simulink model "FIR_TDM_Ex2"  (R2023a)
settings: Solver=VariableStepAuto  StartTime=0.0  StopTime=5  RelTol=1e-3
InitFcn:
  | NumOf_TDM_Channels = 8;
  | SamplesPerChannel = 128;
  | FilterLength = 16;
  | f = dsp.Channelizer(NumOf_TDM_Channels,1,Specification="coefficients");
  | blowpass = firpm(FilterLength-1,[0 .2 .4 1],[1 1 0 0]);
  | N = length(blowpass)-1;
  | Fc = 0.4;
  | j = complex(0,1);
  | bbandpass = blowpass.*exp(j*Fc*pi*(0:N));
  | f.LowpassCoefficients = bbandpass;
  | f.freqz
  | filters = f.getFilters;
  | filters = round(filters, 14, TieBreaker="fromzero");
undefined symbols (not defined in the file): Asymmetric, S, vsva2197, xcvc1902
libraries: aieUtilities x3, dspsrcs4 x2, aieDSP x1, vmcUtilities x1
settings Model: Creator=sdegala  LastModifiedBy=sdegala

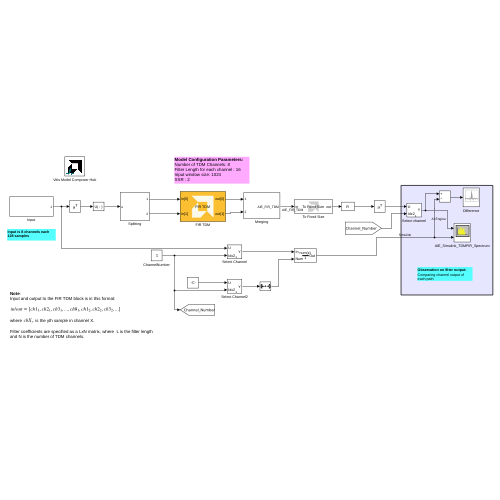
[thumbnail: Simulink's stored preview of the top-level diagram]
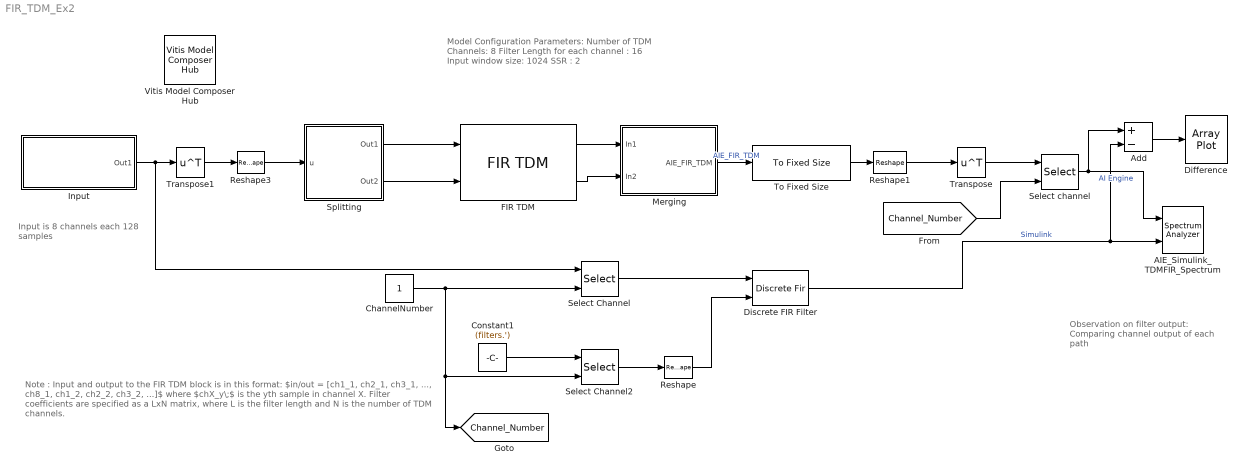
== system FIR_TDM_Ex2 ==
  note: Observation on filter output:
      | Comparing channel output of each path
  note: Input is 8 channels each 128 samples
  note: Model Configuration Parameters:
      | Number of TDM Channels: 8
      | Filter Length for each channel : 16
      | Input window size: 1024
      | SSR : 2
  note: Note :
      | Input and output to the FIR TDM block is in this format:
      |
      | $in/out = [ch1_1, ch2_1, ch3_1, ..., ch8_1, ch1_2, ch2_2, ch3_2, ...]$
      |
      | where $chX_y\;$ is the yth sample in channel X.
      |
      | Filter coefficients are specified as a LxN matrix, where L is the filter length and N is the number of TDM channels.
  AIE_Simulink_TDMFIR_Spectrum : SpectrumAnalyzer  NumInputPorts=2  WindowPosition=[265.000000,-185.000000,936.000000,716.000000,]  Visible=on  ScopeFrameLocation=window  Span=12499.999999999998  StartFrequency=-6249.999999999999  StopFrequency=6249.999999999999  YLimits=[-92.75639585,-29.1140143]  ShowLegend=on  SelectedToolstripTab=spectrumAnalyzerToolstrip.channelMeasurementsTab  MeasurementChannel=2
  Add : Sum  Inputs=+-
  ChannelNumber : Constant  OutDataTypeStr=uint16  SampleTime=-1
  Constant1 : Constant  Value=(filters.')  OutDataTypeStr=single  SampleTime=-1
  Difference : ArrayPlot  WindowPosition=[349.000000,17.000000,800.000000,500.000000,]  Visible=on  ScopeFrameLocation=window  XDataMode=Custom  XOffset=[-0.5 0.5]  PlotType=Line  AxesScaling=Manual  YLimits=[-0.5 0.5]  ShowLegend=on
  Discrete FIR Filter : DiscreteFir  CoefSource=Input port  Coefficients=filters(1,:)  InputProcessing=Columns as channels (frame based)  RndMeth=Round
      settings: InputPortMap=u0,u1
  FIR TDM : aieDSP/FIR TDM  data_type=cfloat  data_out_type=cfloat  coef_type=cfloat  fir_length=FilterLength  coeff=(filters.')  shift_val=0  rnd_mode=Floor  input_window_size=NumOf_TDM_Channels*SamplesPerChannel  tdm_channels=NumOf_TDM_Channels  sat_mode=1-Asymmetric  casc_length=1  ssr=2  AIE_VARIANT=1  blockJsonConstraints=[]  blockJsonConstraintsInternal=[]  spec=vmc_fir_tdm.json  SerializedMaskParamNames=[]  SerializedMaskParamValues=[]  SerializedMaskParamVisibilities=[]  block_type=FIR TDM  SerializedMaskParamDataypes=typename|typename|typename|uint|coef_type|uint|uint|uint|uint|uint|uint|uint|uint  SerializedMaskParamEnumStrArr=0|0|0|0|0|0|Floor,Ceiling,Round to positive infinity,Round to negative infinity,Round symmetrical to infinity,Round symmetrical to zero,Round convergent to even,Round convergent to odd|0|0|0-None,1-Asymmetric,3-Symmetric|0|0|0  SerializedMaskParamEnumValArr=0|0|0|0|0|0|0,1,2,3,4,5,6,7|0|0|0,1,3|0|0|0  SerializedMaskParamVectorArr=0|0|0|0|1|0|0|0|0|0|0|0|0
  Input : Subsystem
  Merging : Subsystem
  Reshape : Reshape  OutputDimensionality=Row vector (2-D)
  Reshape1 : Reshape  OutputDimensionality=Customize  OutputDimensions=[NumOf_TDM_Channels,SamplesPerChannel]
  Reshape3 : Reshape
  Select Channel : Selector  NumberOfDimensions=2  InputPortWidth=3  IndexOptions=Select all,Index vector (port)  Indices=3,[16]  OutputSizes=1,1
  Select Channel2 : Selector  NumberOfDimensions=2  InputPortWidth=3  IndexOptions=Select all,Index vector (port)  Indices=3,[16]  OutputSizes=1,1
  Select channel : Selector  NumberOfDimensions=2  InputPortWidth=3  IndexOptions=Select all,Index vector (port)  Indices=3,[16]  OutputSizes=1,1
  Splitting : Subsystem
  To Fixed Size : aieUtilities/To Fixed Size  Mode=Stop simulation when input variable-size signal is not full  OutputSize=Inherit: Same as input  CopyMethod=Buffer samples to form output  HasStatusOutput=on
  Transpose : Math  Operator=transpose
  Transpose1 : Math  Operator=transpose
  Vitis Model Composer Hub : vmcUtilities/Vitis Model Composer Hub  Tag=genX  CodeGeneration=off  StartColumn=1  NumberOfColumns=1  TargetDirectory=./code  exportDesign=off  analyzeDesign=off  validateDesignOnHw=off  ExportType=AI Engines  IpVendor=xilinx.com  IpLibrary=hls  IpVersion=1.0  IpHWLanguage=Verilog  AieCompilerOptions={}  AieSimulatorOptions={}  CreateTestbench=off  TestbenchStackSize=10  RunRtlSim=off  RunCSim=off  RunAieSim=off  AieSimTimeout=50000  RunAieSimProfiling=off  LaunchVitisAnalyzer=off  PlotOutput=off  RunX86Sim=off  X86SimTimeout=10  GenHwImage=off  GenLibadfXo=off  GenHwValidationCode=off  PlatformType=Not Specified  HwSystemType=Baremetal  HwValidationTarget=hw  ProjDevice=xcvc1902-vsva2197-1LP-e-S  ProjDevicePart=xcvc1902-vsva2197-1LP-e-S  AIEType=AIE  SamplePeriod=-1  ClockFrequency=200  DataPathParallelism=1  xilinxfamily=versalaicore  part=xcvc1902  speed=-1LP-e-S  package=vsva2197  directory=./netlist  testbench=off  incr_netlist=off  synthesis_tool=Vivado  clock_wrapper=Clock Enables  dbl_ovrd=According to Block Masks  dcm_input_clock_period=10  sysclk_period=10  simulink_period=1  eval_field=0  LogFileName=''  NThreads=4
  tag scope: Channel_Number=global
  wires:
  Reshape1/1 -> Transpose/1
  Select channel/1 -> Add/1, AIE_Simulink_TDMFIR_Spectrum/1  "AI Engine"
  Transpose1/1 -> Reshape3/1
  Transpose/1 -> Select channel/1
  Input/1(Out1) -> Transpose1/1, Select Channel/1
  Discrete FIR Filter/1 -> AIE_Simulink_TDMFIR_Spectrum/2, Add/2  "Simulink"
  Select Channel/1 -> Discrete FIR Filter/1
  Reshape3/1 -> Splitting/1(u)
  Splitting/1(Out1) -> FIR TDM/1
  Splitting/2(Out2) -> FIR TDM/2
  Merging/1(AIE_FIR_TDM) -> To Fixed Size/1  "AIE_FIR_TDM"
  FIR TDM/1 -> Merging/1(In1)
  FIR TDM/2 -> Merging/2(In2)
  To Fixed Size/1 -> Reshape1/1
  ChannelNumber/1 -> Select Channel2/2, [Channel_Number], Select Channel/2
  [Channel_Number] -> Select channel/2
  Add/1 -> Difference/1
  Constant1/1 -> Select Channel2/1
  Select Channel2/1 -> Reshape/1
  Reshape/1 -> Discrete FIR Filter/2

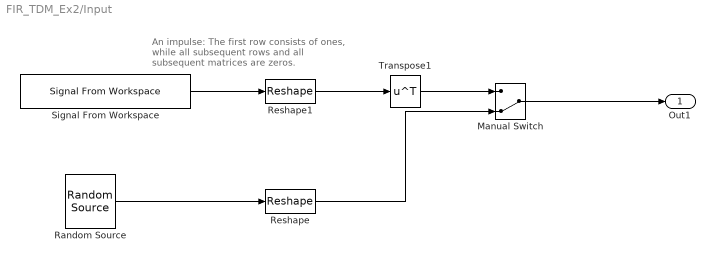
== system FIR_TDM_Ex2/Input ==
  note: An impulse: The first row consists of ones,
      | while all subsequent rows and all subsequent matrices are zeros.
  Manual Switch : ManualSwitch  CurrentSetting=0
  Random Source : dspsrcs4/Random Source  SrcType=Gaussian  NormMethod=Ziggurat  CltLength=12  MinVal=0  MaxVal=1  MeanVal=0  VarVal=1e-4  RepMode=Specify seed  rawSeed=1  IsInherit=off  SampMode=Discrete  SampTime=1/100e3  SampFrame=SamplesPerChannel*NumOf_TDM_Channels  DataType=Single  OutComplex=Complex  OutputFrames=on
  Reshape : Reshape  OutputDimensionality=Customize  OutputDimensions=[SamplesPerChannel,NumOf_TDM_Channels]
  Reshape1 : Reshape  OutputDimensionality=Customize  OutputDimensions=[NumOf_TDM_Channels,SamplesPerChannel]
  Signal From Workspace : dspsrcs4/Signal From Workspace  X=single(complex(ones(1,NumOf_TDM_Channels)))  Ts=1/100e3  nsamps=SamplesPerChannel*NumOf_TDM_Channels  OutputAfterFinalValue=Setting to zero  ignoreOrWarnInputAndFrameLengths=off  OutputFrames=off
  Transpose1 : Math  Operator=transpose
  Out1 : Outport
  wires:
  Manual Switch/1 -> Out1/1
  Random Source/1 -> Reshape/1
  Signal From Workspace/1 -> Reshape1/1
  Reshape/1 -> Manual Switch/2
  Reshape1/1 -> Transpose1/1
  Transpose1/1 -> Manual Switch/1

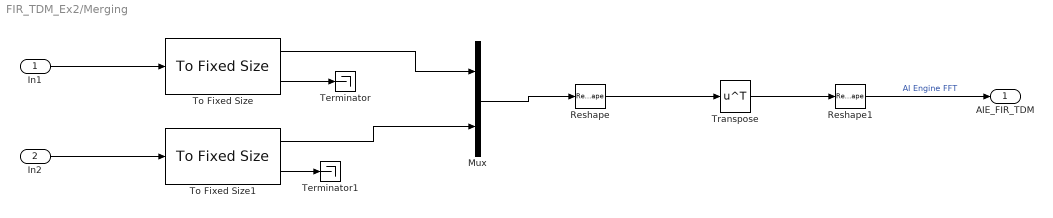
== system FIR_TDM_Ex2/Merging ==
  In1 : Inport
  In2 : Inport  Port=2
  Mux : Mux  Inputs=2
  Reshape : Reshape  OutputDimensionality=Customize  OutputDimensions=[512, 2]
  Reshape1 : Reshape  OutputDimensions=[1, 10]
  Terminator : Terminator
  Terminator1 : Terminator
  To Fixed Size : aieUtilities/To Fixed Size  Mode=Produce a valid output signal  OutputSize=Inherit: Same as input  CopyMethod=Buffer samples to form output  HasStatusOutput=on
  To Fixed Size1 : aieUtilities/To Fixed Size  Mode=Produce a valid output signal  OutputSize=Inherit: Same as input  CopyMethod=Buffer samples to form output  HasStatusOutput=on
  Transpose : Math  Operator=transpose
  AIE_FIR_TDM : Outport
  wires:
  Reshape/1 -> Transpose/1
  To Fixed Size1/2 -> Terminator1/1
  To Fixed Size1/1 -> Mux/2
  In2/1 -> To Fixed Size1/1
  To Fixed Size/2 -> Terminator/1
  Transpose/1 -> Reshape1/1
  To Fixed Size/1 -> Mux/1
  Mux/1 -> Reshape/1
  Reshape1/1 -> AIE_FIR_TDM/1  "AI Engine FFT"
  In1/1 -> To Fixed Size/1

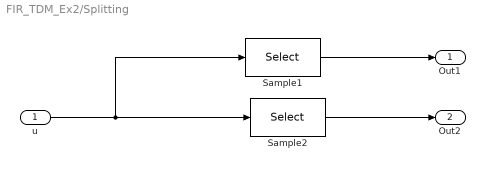
== system FIR_TDM_Ex2/Splitting ==
  u : Inport
  Sample1 : Selector  InputPortWidth=1024  IndexOptions=Index vector (dialog)  Indices=1:2:1024  OutputSizes=1
  Sample2 : Selector  InputPortWidth=1024  IndexOptions=Index vector (dialog)  Indices=2:2:1024  OutputSizes=1
  Out1 : Outport
  Out2 : Outport  Port=2
  wires:
  u/1 -> Sample2/1, Sample1/1
  Sample2/1 -> Out2/1
  Sample1/1 -> Out1/1
